simulink model "SimulationDemo_Ship"  (R2025a)
settings: Solver=ode4  StartTime=0.0  StopTime=200  FixedStep=0.02  RelTol=1e-3
InitFcn:
  | Initialization
model workspace (MAT data in the model file):
  actuatorInitial : object (value not decoded)
  contactParams : object (value not decoded)
  flightProtection : object (value not decoded)
  initial : object (value not decoded)
symbols that are objects in the model workspace (value not decoded): actuatorInitial, contactParams, flightProtection, initial
undefined symbols (not defined in the file): aeroData, aileronMax, aileronMin, dirPitch, dirRoll, dirThrottle, dirYaw, elevatorMax, elevatorMin, envCatalog, F, geometry, Light, MIL, pitchCh, pitchDB, propulsionData, rollCh, rollDB, rudderMax, rudderMin, throttleCh, throttleDB, uPitchMax, uPitchMin, uRollMax, uRollMin, uThrottleMax, uThrottleMin, uYawMax, uYawMin, yawCh, yawDB
libraries: simulink_extras x4, aerolibwind2 x3, aerolibasang x2, aerolibsim3d x2, aerolibadyn x1, matrix_library x1, aerolibanimutils x1, aerolibatmos2 x1, uavutilslib x1, sim3dlib x1
(part 2 of 2)

== system SimulationDemo_Ship/Aircraft Dynamics/Forces & Moments/Aerodynamic Forces & Moments/Elevator Contribution ==
  Elevator : Inport
  Alpha : Inport  Port=2
  Bus Creator : BusCreator  Inputs=3
  CD Lookup : Lookup_n-D  LookupTableObject=k  BreakpointsForDimension1=aeroData.elevatorData.ControlDeflections  BreakpointsForDimension2=aeroData.elevatorData.Alpha  Table=aeroData.elevatorData.CD  InternalRulePriority=Speed  RndMeth=Simplest
      settings: InputPortMap=u0,u1
  "CL Lookup " : Lookup_n-D  BreakpointsForDimension1=aeroData.elevatorData.ControlDeflections  BreakpointsForDimension2=aeroData.elevatorData.Alpha  Table=aeroData.elevatorData.CL  InternalRulePriority=Speed  RndMeth=Simplest
      settings: InputPortMap=u0,u1
  Cm Lookup : Lookup_n-D  BreakpointsForDimension1=aeroData.elevatorData.ControlDeflections  BreakpointsForDimension2=aeroData.elevatorData.Alpha  Table=aeroData.elevatorData.Cm  InternalRulePriority=Speed  RndMeth=Simplest
      settings: InputPortMap=u0,u1
  Elevator Contribution : Outport
  wires:
  Bus Creator/1 -> Elevator Contribution/1
  Alpha/1 -> Cm Lookup/2, "CL Lookup "/2, CD Lookup/2
  Elevator/1 -> "CL Lookup "/1, Cm Lookup/1, CD Lookup/1
  Cm Lookup/1 -> Bus Creator/3  "Cm"
  CD Lookup/1 -> Bus Creator/1  "CD"
  "CL Lookup "/1 -> Bus Creator/2  "CL"

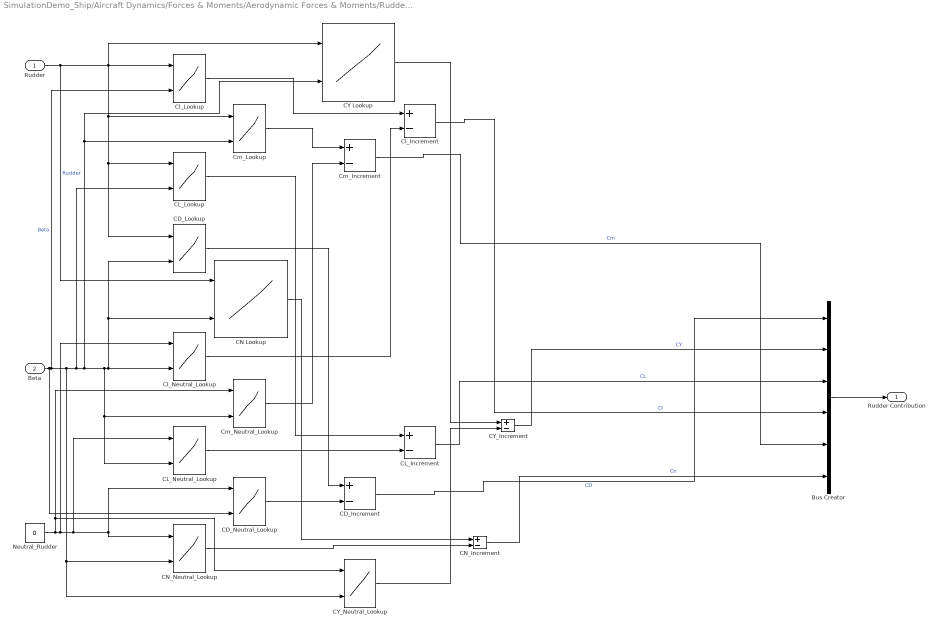
== system SimulationDemo_Ship/Aircraft Dynamics/Forces & Moments/Aerodynamic Forces & Moments/Rudder Contribution ==
  Rudder : Inport
  Beta : Inport  Port=2
  Bus Creator : BusCreator  Inputs=6
  CD_Increment : Sum  Inputs=+-
  CD_Lookup : Lookup_n-D  BreakpointsForDimension1=aeroData.rudderData.ControlDeflections  BreakpointsForDimension2=aeroData.rudderData.Beta  Table=aeroData.rudderData.CD
      settings: InputPortMap=u0,u1
  CD_Neutral_Lookup : Lookup_n-D  BreakpointsForDimension1=aeroData.rudderData.ControlDeflections  BreakpointsForDimension2=aeroData.rudderData.Beta  Table=aeroData.rudderData.CD
      settings: InputPortMap=u0,u1
  CL_Increment : Sum  Inputs=+-
  CL_Lookup : Lookup_n-D  BreakpointsForDimension1=aeroData.rudderData.ControlDeflections  BreakpointsForDimension2=aeroData.rudderData.Beta  Table=aeroData.rudderData.CL
      settings: InputPortMap=u0,u1
  CL_Neutral_Lookup : Lookup_n-D  BreakpointsForDimension1=aeroData.rudderData.ControlDeflections  BreakpointsForDimension2=aeroData.rudderData.Beta  Table=aeroData.rudderData.CL
      settings: InputPortMap=u0,u1
  "CN Lookup " : Lookup_n-D  BreakpointsForDimension1=aeroData.rudderData.ControlDeflections  BreakpointsForDimension2=aeroData.rudderData.Beta  Table=aeroData.rudderData.Cn  InternalRulePriority=Speed  RndMeth=Simplest
      settings: InputPortMap=u0,u1
  CN_Increment : Sum  Inputs=+-
  CN_Neutral_Lookup : Lookup_n-D  BreakpointsForDimension1=aeroData.rudderData.ControlDeflections  BreakpointsForDimension2=aeroData.rudderData.Beta  Table=aeroData.rudderData.Cn
      settings: InputPortMap=u0,u1
  CY Lookup : Lookup_n-D  BreakpointsForDimension1=aeroData.rudderData.ControlDeflections  BreakpointsForDimension2=aeroData.rudderData.Beta  Table=aeroData.rudderData.CY  InternalRulePriority=Speed  RndMeth=Simplest
      settings: InputPortMap=u0,u1
  CY_Increment : Sum  Inputs=+-
  CY_Neutral_Lookup : Lookup_n-D  BreakpointsForDimension1=aeroData.rudderData.ControlDeflections  BreakpointsForDimension2=aeroData.rudderData.Beta  Table=aeroData.rudderData.CY
      settings: InputPortMap=u0,u1
  Cl_Increment : Sum  Inputs=+-
  Cl_Lookup : Lookup_n-D  BreakpointsForDimension1=aeroData.rudderData.ControlDeflections  BreakpointsForDimension2=aeroData.rudderData.Beta  Table=aeroData.rudderData.Cl
      settings: InputPortMap=u0,u1
  Cl_Neutral_Lookup : Lookup_n-D  BreakpointsForDimension1=aeroData.rudderData.ControlDeflections  BreakpointsForDimension2=aeroData.rudderData.Beta  Table=aeroData.rudderData.Cl
      settings: InputPortMap=u0,u1
  Cm_Increment : Sum  Inputs=+-
  Cm_Lookup : Lookup_n-D  BreakpointsForDimension1=aeroData.rudderData.ControlDeflections  BreakpointsForDimension2=aeroData.rudderData.Beta  Table=aeroData.rudderData.Cm
      settings: InputPortMap=u0,u1
  Cm_Neutral_Lookup : Lookup_n-D  BreakpointsForDimension1=aeroData.rudderData.ControlDeflections  BreakpointsForDimension2=aeroData.rudderData.Beta  Table=aeroData.rudderData.Cm
      settings: InputPortMap=u0,u1
  Neutral_Rudder : Constant  Value=0
  "Rudder Contribution " : Outport
  wires:
  Cm_Neutral_Lookup/1 -> Cm_Increment/2
  Cm_Lookup/1 -> Cm_Increment/1
  Cl_Neutral_Lookup/1 -> Cl_Increment/2
  Cl_Lookup/1 -> Cl_Increment/1
  CL_Neutral_Lookup/1 -> CL_Increment/2
  CL_Lookup/1 -> CL_Increment/1
  CD_Neutral_Lookup/1 -> CD_Increment/2
  CD_Lookup/1 -> CD_Increment/1
  Rudder/1 -> CD_Lookup/1, CL_Lookup/1, Cm_Lookup/1, CY Lookup/1, Cl_Lookup/1, "CN Lookup "/1  "Rudder"
  Beta/1 -> CY_Neutral_Lookup/2, CN_Neutral_Lookup/2, CL_Neutral_Lookup/2, Cm_Neutral_Lookup/2, "CN Lookup "/2, CD_Lookup/2, Cl_Neutral_Lookup/2, CY Lookup/2, Cm_Lookup/2, CL_Lookup/2, Cl_Lookup/2, CD_Neutral_Lookup/2  "Beta"
  Neutral_Rudder/1 -> CN_Neutral_Lookup/1, CD_Neutral_Lookup/1, CL_Neutral_Lookup/1, Cl_Neutral_Lookup/1, CY_Neutral_Lookup/1, Cm_Neutral_Lookup/1
  CY Lookup/1 -> CY_Increment/1
  CY_Neutral_Lookup/1 -> CY_Increment/2
  "CN Lookup "/1 -> CN_Increment/1
  CN_Neutral_Lookup/1 -> CN_Increment/2
  Cl_Increment/1 -> Bus Creator/4  "Cl"
  CD_Increment/1 -> Bus Creator/1  "CD"
  Cm_Increment/1 -> Bus Creator/5  "Cm"
  CY_Increment/1 -> Bus Creator/2  "CY"
  CL_Increment/1 -> Bus Creator/3  "CL"
  Bus Creator/1 -> "Rudder Contribution "/1
  CN_Increment/1 -> Bus Creator/6  "Cn"

== system SimulationDemo_Ship/Aircraft Dynamics/Forces & Moments/Aerodynamic Forces & Moments/Subsystem ==
  Elevator contributiotion : Inport
  Aileron contributiotion : Inport  Port=2
  Rudder contributiotion : Inport  Port=3
  Damping rate contributions : Inport  Port=4
  Bus Selector : BusSelector  OutputSignals=CD,CL,Cm
  Bus Selector1 : BusSelector  OutputSignals=CD,CY,CL,Cl,Cm,Cn
  Bus Selector2 : BusSelector  OutputSignals=CD,CY,CL,Cl,Cm,Cn
  Bus Selector3 : BusSelector  OutputSignals=CD_rate,CY_rate,CL_rate,Cl_damp,Cm_damp,Cn_damp
  CD_Total : Sum  Inputs=++++
  CL_Total : Sum  Inputs=++++
  CY_Total : Sum  Inputs=+++
  Cl_Base_Total : Sum  Inputs=+++
  Cm_Base_Total : Sum  Inputs=++++
  Cn_Base_Total : Sum  Inputs=+++
  Moment coefficients : Mux  Inputs=3
  Mux : Mux  Inputs=3
  Forces Coefficients : Outport
  Moment Coefficients : Outport  Port=2
  wires:
  Bus Selector3/2 -> CY_Total/3  "<CY_rate>"
  Bus Selector2/3 -> CL_Total/3  "<CL>"
  Elevator contributiotion/1 -> Bus Selector/1
  CL_Total/1 -> Mux/3  "CL_Total"
  Aileron contributiotion/1 -> Bus Selector1/1
  Cn_Base_Total/1 -> Moment coefficients/3
  Rudder contributiotion/1 -> Bus Selector2/1
  Bus Selector1/1 -> CD_Total/2  "<CD>"
  Damping rate contributions/1 -> Bus Selector3/1
  Bus Selector/1 -> CD_Total/1  "<CD>"
  Bus Selector/2 -> CL_Total/1  "<CL>"
  Bus Selector2/1 -> CD_Total/3  "<CD>"
  Bus Selector/3 -> Cm_Base_Total/1  "<Cm>"
  Bus Selector1/2 -> CY_Total/1  "<CY>"
  CY_Total/1 -> Mux/2  "CY_Total"
  Bus Selector1/3 -> CL_Total/2  "<CL>"
  Bus Selector1/4 -> Cl_Base_Total/1  "<Cl>"
  Bus Selector1/5 -> Cm_Base_Total/2  "<Cm>"
  Mux/1 -> Forces Coefficients/1
  Bus Selector1/6 -> Cn_Base_Total/1  "<Cn>"
  Bus Selector2/2 -> CY_Total/2  "<CY>"
  Bus Selector2/4 -> Cl_Base_Total/2  "<Cl>"
  Bus Selector2/5 -> Cm_Base_Total/3  "<Cm>"
  Bus Selector2/6 -> Cn_Base_Total/2  "<Cn>"
  Bus Selector3/1 -> CD_Total/4  "<CD_rate>"
  Bus Selector3/3 -> CL_Total/4  "<CL_rate>"
  Bus Selector3/4 -> Cl_Base_Total/3  "<Cl_damp>"
  Bus Selector3/5 -> Cm_Base_Total/4  "<Cm_damp>"
  Bus Selector3/6 -> Cn_Base_Total/3  "<Cn_damp>"
  CD_Total/1 -> Mux/1  "CD_Total"
  Cl_Base_Total/1 -> Moment coefficients/1
  Cm_Base_Total/1 -> Moment coefficients/2
  Moment coefficients/1 -> Moment Coefficients/1

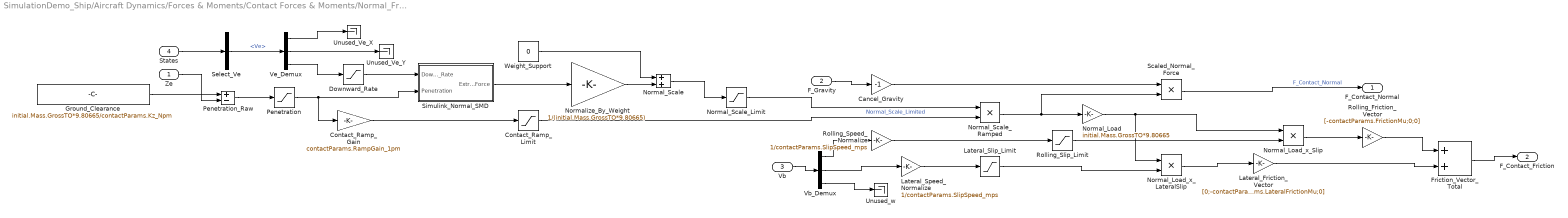
== system SimulationDemo_Ship/Aircraft Dynamics/Forces & Moments/Contact Forces & Moments/Normal_Friction_Forces ==
  Ze : Inport
  F_Gravity : Inport  Port=2
  Vb : Inport  Port=3
  States : Inport  Port=4
  Cancel_Gravity : Gain  Gain=-1
  Contact_Ramp_Gain : Gain  Gain=contactParams.RampGain_1pm
  Contact_Ramp_Limit : Saturate  UpperLimit=1  LowerLimit=0
  Downward_Rate : Saturate  UpperLimit=inf  LowerLimit=-inf
  Friction_Vector_Total : Sum
  Ground_Clearance : Constant  Value=initial.Mass.GrossTO*9.80665/contactParams.Kz_Npm
  Lateral_Friction_Vector : Gain  Gain=[0;-contactParams.LateralFrictionMu;0]
  Lateral_Slip_Limit : Saturate  UpperLimit=1  LowerLimit=-1
  Lateral_Speed_Normalize : Gain  Gain=1/contactParams.SlipSpeed_mps
  Normal_Load : Gain  Gain=initial.Mass.GrossTO*9.80665
  Normal_Load_x_LateralSlip : Product
  Normal_Load_x_Slip : Product
  Normal_Scale : Sum
  Normal_Scale_Limit : Saturate  UpperLimit=contactParams.NormalScaleMax  LowerLimit=0
  Normal_Scale_Ramped : Product
  Normalize_By_Weight : Gain  Gain=1/(initial.Mass.GrossTO*9.80665)
  Penetration : Saturate  UpperLimit=inf  LowerLimit=0
  Penetration_Raw : Sum  Inputs=+-
  Rolling_Friction_Vector : Gain  Gain=[-contactParams.FrictionMu;0;0]
  Rolling_Slip_Limit : Saturate  UpperLimit=1  LowerLimit=-1
  Rolling_Speed_Normalize : Gain  Gain=1/contactParams.SlipSpeed_mps
  Scaled_Normal_Force : Product
  Select_Ve : BusSelector  OutputSignals=Ve
  Simulink_Normal_SMD : Subsystem
  Unused_Ve_X : Terminator
  Unused_Ve_Y : Terminator
  Unused_w : Terminator
  Vb_Demux : Demux  Outputs=3
  Ve_Demux : Demux  Outputs=3
  Weight_Support : Constant  Value=0
  F_Contact_Normal : Outport
  F_Contact_Friction : Outport  Port=2
  wires:
  Friction_Vector_Total/1 -> F_Contact_Friction/1
  Lateral_Friction_Vector/1 -> Friction_Vector_Total/2
  Rolling_Friction_Vector/1 -> Friction_Vector_Total/1
  Normal_Load_x_LateralSlip/1 -> Lateral_Friction_Vector/1
  Lateral_Slip_Limit/1 -> Normal_Load_x_LateralSlip/2
  Lateral_Speed_Normalize/1 -> Lateral_Slip_Limit/1
  Vb_Demux/2 -> Lateral_Speed_Normalize/1
  Normalize_By_Weight/1 -> Normal_Scale/2
  Penetration/1 -> Simulink_Normal_SMD/2(Penetration), Contact_Ramp_Gain/1
  Rolling_Slip_Limit/1 -> Normal_Load_x_Slip/2
  Normal_Scale_Ramped/1 -> Normal_Load/1, Scaled_Normal_Force/2
  Ze/1 -> Penetration_Raw/2
  Contact_Ramp_Limit/1 -> Normal_Scale_Ramped/2
  Ground_Clearance/1 -> Penetration_Raw/1
  Normal_Scale_Limit/1 -> Normal_Scale_Ramped/1  "Normal_Scale_Limited"
  Contact_Ramp_Gain/1 -> Contact_Ramp_Limit/1
  Downward_Rate/1 -> Simulink_Normal_SMD/1(Downward_Rate)
  Penetration_Raw/1 -> Penetration/1
  Scaled_Normal_Force/1 -> F_Contact_Normal/1  "F_Contact_Normal"
  Normal_Load/1 -> Normal_Load_x_Slip/1, Normal_Load_x_LateralSlip/1
  F_Gravity/1 -> Cancel_Gravity/1
  Normal_Scale/1 -> Normal_Scale_Limit/1
  Simulink_Normal_SMD/1(Extra_Normal_Force) -> Normalize_By_Weight/1
  Vb_Demux/1 -> Rolling_Speed_Normalize/1
  Weight_Support/1 -> Normal_Scale/1
  Cancel_Gravity/1 -> Scaled_Normal_Force/1
  Vb/1 -> Vb_Demux/1
  Rolling_Speed_Normalize/1 -> Rolling_Slip_Limit/1
  Normal_Load_x_Slip/1 -> Rolling_Friction_Vector/1
  Vb_Demux/3 -> Unused_w/1
  States/1 -> Select_Ve/1
  Select_Ve/1 -> Ve_Demux/1  "<Ve>"
  Ve_Demux/1 -> Unused_Ve_X/1
  Ve_Demux/2 -> Unused_Ve_Y/1
  Ve_Demux/3 -> Downward_Rate/1

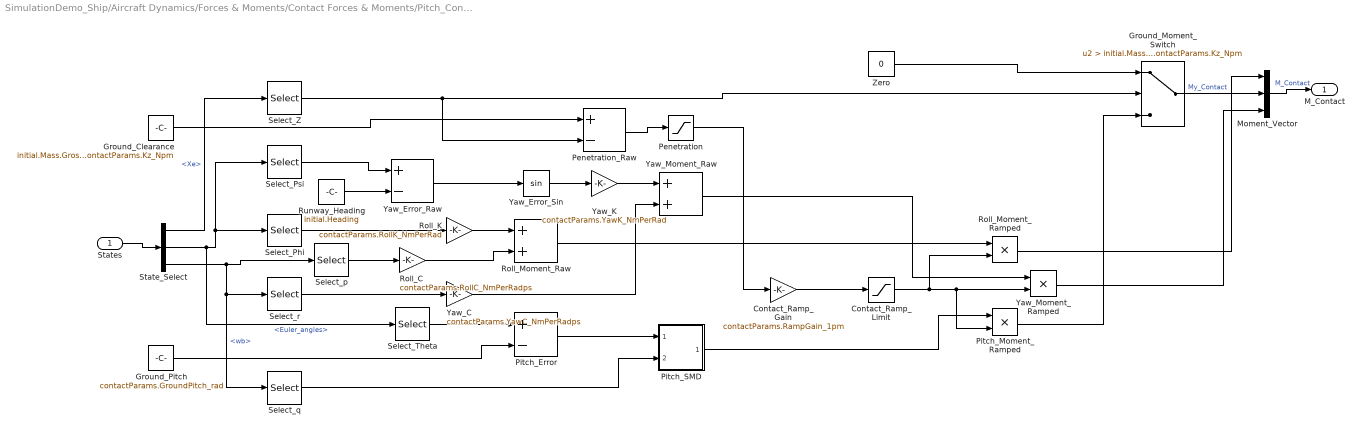
== system SimulationDemo_Ship/Aircraft Dynamics/Forces & Moments/Contact Forces & Moments/Pitch_Contact_Moment ==
  States : Inport
  Contact_Ramp_Gain : Gain  Gain=contactParams.RampGain_1pm
  Contact_Ramp_Limit : Saturate  UpperLimit=1  LowerLimit=0
  Ground_Clearance : Constant  Value=initial.Mass.GrossTO*9.80665/contactParams.Kz_Npm
  Ground_Moment_Switch : Switch  Criteria=u2 > Threshold  Threshold=initial.Mass.GrossTO*9.80665/contactParams.Kz_Npm
  Ground_Pitch : Constant  Value=contactParams.GroundPitch_rad
  Moment_Vector : Mux  Inputs=3
  Penetration : Saturate  UpperLimit=inf  LowerLimit=0
  Penetration_Raw : Sum  Inputs=+-
  Pitch_Error : Sum  Inputs=+-
  Pitch_Moment_Ramped : Product
  Pitch_SMD : Subsystem
  Roll_C : Gain  Gain=contactParams.RollC_NmPerRadps
  Roll_K : Gain  Gain=contactParams.RollK_NmPerRad
  Roll_Moment_Ramped : Product
  Roll_Moment_Raw : Sum
  Runway_Heading : Constant  Value=initial.Heading
  Select_Phi : Selector  InputPortWidth=3  IndexOptions=Index vector (dialog)  Indices=1  OutputSizes=1
  Select_Psi : Selector  InputPortWidth=3  IndexOptions=Index vector (dialog)  Indices=3  OutputSizes=1
  Select_Theta : Selector  InputPortWidth=3  IndexOptions=Index vector (dialog)  Indices=[2]  OutputSizes=1
  Select_Z : Selector  InputPortWidth=3  IndexOptions=Index vector (dialog)  Indices=[3]  OutputSizes=1
  Select_p : Selector  InputPortWidth=3  IndexOptions=Index vector (dialog)  Indices=1  OutputSizes=1
  Select_q : Selector  InputPortWidth=3  IndexOptions=Index vector (dialog)  Indices=[2]  OutputSizes=1
  Select_r : Selector  InputPortWidth=3  IndexOptions=Index vector (dialog)  Indices=3  OutputSizes=1
  State_Select : BusSelector  OutputSignals=Xe,Euler_angles,wb
  Yaw_C : Gain  Gain=contactParams.YawC_NmPerRadps
  Yaw_Error_Raw : Sum  Inputs=+-
  Yaw_Error_Sin : Trigonometry
  Yaw_K : Gain  Gain=contactParams.YawK_NmPerRad
  Yaw_Moment_Ramped : Product
  Yaw_Moment_Raw : Sum
  Zero : Constant  Value=0
  M_Contact : Outport
  wires:
  Yaw_Moment_Ramped/1 -> Moment_Vector/3
  Roll_Moment_Ramped/1 -> Moment_Vector/1
  Yaw_Moment_Raw/1 -> Yaw_Moment_Ramped/1
  Yaw_C/1 -> Yaw_Moment_Raw/2
  Yaw_K/1 -> Yaw_Moment_Raw/1
  Select_r/1 -> Yaw_C/1
  Yaw_Error_Sin/1 -> Yaw_K/1
  Yaw_Error_Raw/1 -> Yaw_Error_Sin/1
  Runway_Heading/1 -> Yaw_Error_Raw/2
  Select_Psi/1 -> Yaw_Error_Raw/1
  Roll_Moment_Raw/1 -> Roll_Moment_Ramped/1
  Roll_C/1 -> Roll_Moment_Raw/2
  Roll_K/1 -> Roll_Moment_Raw/1
  Select_p/1 -> Roll_C/1
  Select_Phi/1 -> Roll_K/1
  States/1 -> State_Select/1
  State_Select/1 -> Select_Z/1  "<Xe>"
  State_Select/2 -> Select_Phi/1, Select_Psi/1, Select_Theta/1  "<Euler_angles>"
  State_Select/3 -> Select_q/1, Select_r/1, Select_p/1  "<wb>"
  Ground_Clearance/1 -> Penetration_Raw/1
  Select_Z/1 -> Ground_Moment_Switch/2, Penetration_Raw/2
  Penetration_Raw/1 -> Penetration/1
  Penetration/1 -> Contact_Ramp_Gain/1
  Contact_Ramp_Gain/1 -> Contact_Ramp_Limit/1
  Select_Theta/1 -> Pitch_Error/1
  Ground_Pitch/1 -> Pitch_Error/2
  Pitch_Error/1 -> Pitch_SMD/1(Pitch_Error)
  Select_q/1 -> Pitch_SMD/2(Pitch_Rate)
  Pitch_SMD/1(Pitch_Moment) -> Pitch_Moment_Ramped/1
  Contact_Ramp_Limit/1 -> Pitch_Moment_Ramped/2, Yaw_Moment_Ramped/2, Roll_Moment_Ramped/2
  Zero/1 -> Ground_Moment_Switch/1
  Pitch_Moment_Ramped/1 -> Ground_Moment_Switch/3
  Ground_Moment_Switch/1 -> Moment_Vector/2  "My_Contact"
  Moment_Vector/1 -> M_Contact/1  "M_Contact"

== system SimulationDemo_Ship/Aircraft Dynamics/Forces & Moments/Propulsion Forces & Moments/Density Correction ==
  In1 : Inport
  Bus Selector1 : BusSelector  OutputSignals=rho
  Constant : Constant  Value=1.225
  Divide : Product  Inputs=*/
  Out1 : Outport
  wires:
  Bus Selector1/1 -> Divide/1  "<rho>"
  Divide/1 -> Out1/1
  Constant/1 -> Divide/2
  In1/1 -> Bus Selector1/1

== system SimulationDemo_Ship/Aircraft Dynamics/Forces & Moments/Propulsion Forces & Moments/Subsystem ==
  Forces : Inport
  Cross Product : matrix_library/Cross Product
  Position Vector : Concatenate  NumInputs=3  ConcatenateDimension=2
  Thrust Vector : Concatenate  NumInputs=1  Mode=Multidimensional array  ConcatenateDimension=3
  rX : Constant  Value=geometry.PropArmX
  rY : Constant  Value=geometry.PropArmY
  rZ : Constant  Value=geometry.PropArmZ
  Moments : Outport
  wires:
  rZ/1 -> Position Vector/3
  rY/1 -> Position Vector/2
  rX/1 -> Position Vector/1
  Forces/1 -> Thrust Vector/1
  Cross Product/1 -> Moments/1
  Position Vector/1 -> Cross Product/1
  Thrust Vector/1 -> Cross Product/2

== system SimulationDemo_Ship/Aircraft Dynamics/Forces & Moments/Propulsion Forces & Moments/Subsystem1 ==
  Density corrected Thrust : Inport
  Constant : Constant  Value=0
  Cos : Trigonometry  Operator=cos
  Gain : Gain  Gain=-1
  Mux : Mux  Inputs=3
  Product : Product
  Product1 : Product
  Sin : Trigonometry
  Thrust Incidence : Constant  Value=geometry.ThrustIncidence_deg*pi/180
  Forces_Propulsion : Outport
  wires:
  Gain/1 -> Mux/3  "Thrust Z"
  Cos/1 -> Product/2
  Product/1 -> Mux/1  "Thrust X"
  Density corrected Thrust/1 -> Product1/1, Product/1
  Thrust Incidence/1 -> Sin/1, Cos/1
  Sin/1 -> Product1/2
  Product1/1 -> Gain/1
  Constant/1 -> Mux/2  "Thrust Y"
  Mux/1 -> Forces_Propulsion/1  "Forces_Propulsion"

== system SimulationDemo_Ship/Aircraft Dynamics/Forces & Moments/Propulsion Forces & Moments/Subsystem2 ==
  Pilot_Inputs : Inport
  Bus Selector : BusSelector  OutputSignals=Throttle
  Inv_Thrust_Tau : Gain  Gain=5
  Thrust : Lookup_n-D  NumberOfTableDimensions=1  BreakpointsForDimension1=propulsionData.Throttle  IndexSearchMethod=Evenly spaced points  Table=propulsionData.Thrust_Newtons  InternalRulePriority=Speed  RndMeth=Simplest
  Thrust_Lag : Integrator
  Thrust_Lag_Error : Sum  Inputs=+-
  Thrust_Rate_Limiter : RateLimiter  RisingSlewLimit=max(propulsionData.Thrust_Newtons(:))/0.2  FallingSlewLimit=-max(propulsionData.Thrust_Newtons(:))/0.2
  Motor_Prop_Thrust : Outport
  wires:
  Bus Selector/1 -> Thrust/1  "<Throttle>"
  Inv_Thrust_Tau/1 -> Thrust_Lag/1
  Thrust_Lag_Error/1 -> Inv_Thrust_Tau/1
  Thrust_Lag/1 -> Thrust_Lag_Error/2, Motor_Prop_Thrust/1  "Motor_Prop_Thrust"
  Pilot_Inputs/1 -> Bus Selector/1
  Thrust/1 -> Thrust_Rate_Limiter/1  "Static_Thrust"
  Thrust_Rate_Limiter/1 -> Thrust_Lag_Error/1  "Rate_Limited_Thrust"

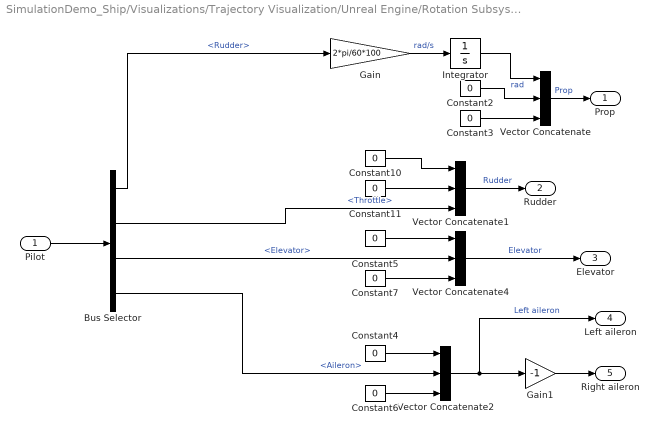
== system SimulationDemo_Ship/Visualizations/Trajectory Visualization/Unreal Engine/Rotation Subsystem ==
  Pilot : Inport
  Bus Selector : BusSelector  OutputSignals=Rudder,Throttle,Elevator,Aileron
  Constant{2..7,10..11} (8 alike) : Constant  Value=0
  Gain : Gain  Gain=2*pi/60*100
  Gain1 : Gain  Gain=-1
  Integrator : Integrator
  Vector Concatenate{,1..2,4} (4 alike) : Concatenate  NumInputs=3  Mode=Multidimensional array  ConcatenateDimension=2
  Prop : Outport  Unit=rad  PortDimensions=[1,3]
  Rudder : Outport  Port=2  Unit=rad  PortDimensions=[1,3]
  Elevator : Outport  Port=3  Unit=rad  PortDimensions=[1,3]
  Left aileron : Outport  Port=4  Unit=rad  PortDimensions=[1,3]
  Right aileron : Outport  Port=5  Unit=rad  PortDimensions=[1,3]
  wires:
  Constant6/1 -> Vector Concatenate2/3
  Constant4/1 -> Vector Concatenate2/1
  Gain1/1 -> Right aileron/1
  Constant11/1 -> Vector Concatenate1/2
  Constant10/1 -> Vector Concatenate1/1
  Constant5/1 -> Vector Concatenate4/1
  Pilot/1 -> Bus Selector/1
  Bus Selector/2 -> Vector Concatenate1/3  "<Throttle>"
  Constant3/1 -> Vector Concatenate/3
  Bus Selector/4 -> Vector Concatenate2/2  "<Aileron>"
  Bus Selector/3 -> Vector Concatenate4/2  "<Elevator>"
  Bus Selector/1 -> Gain/1  "<Rudder>"
  Constant7/1 -> Vector Concatenate4/3
  Vector Concatenate1/1 -> Rudder/1  "Rudder"
  Integrator/1 -> Vector Concatenate/1  "rad"
  Vector Concatenate2/1 -> Gain1/1, Left aileron/1  "Left aileron"
  Vector Concatenate4/1 -> Elevator/1  "Elevator"
  Gain/1 -> Integrator/1  "rad/s"
  Constant2/1 -> Vector Concatenate/2
  Vector Concatenate/1 -> Prop/1  "Prop"

== system SimulationDemo_Ship/Aircraft Dynamics/Forces & Moments/Aerodynamic Forces & Moments/Damping rate coefficients/Cl ==
  p_nd : Inport
  beta : Inport  Port=2
  r_nd : Inport  Port=3
  Constant : Constant  Value=aeroData.stabilityDerivatives.Clp
  Constant1 : Constant  Value=aeroData.stabilityDerivatives.Clr
  Constant2 : Constant  Value=aeroData.stabilityDerivatives.Clb
  Product : Product
  Product1 : Product
  Product2 : Product
  Sum : Sum  Inputs=|+++
  Cl_damp : Outport  VectorParamsAs1DForOutWhenUnconnected=off
  wires:
  Product2/1 -> Sum/3
  Product/1 -> Sum/1
  Constant/1 -> Product/1
  Constant2/1 -> Product1/1
  p_nd/1 -> Product/2
  beta/1 -> Product1/2
  Product1/1 -> Sum/2
  Constant1/1 -> Product2/1
  Sum/1 -> Cl_damp/1
  r_nd/1 -> Product2/2

== system SimulationDemo_Ship/Aircraft Dynamics/Forces & Moments/Aerodynamic Forces & Moments/Damping rate coefficients/Cm ==
  q_nd : Inport
  Constant : Constant  Value=aeroData.stabilityDerivatives.Cmq
  Product : Product
  Cm_damp : Outport
  wires:
  Constant/1 -> Product/1
  q_nd/1 -> Product/2
  Product/1 -> Cm_damp/1  "Cm_damp"

== system SimulationDemo_Ship/Aircraft Dynamics/Forces & Moments/Aerodynamic Forces & Moments/Damping rate coefficients/Cn ==
  p_nd : Inport
  beta : Inport  Port=2
  r_nd : Inport  Port=3
  Constant : Constant  Value=aeroData.stabilityDerivatives.Cnp
  Constant1 : Constant  Value=aeroData.stabilityDerivatives.Cnr
  Constant2 : Constant  Value=aeroData.stabilityDerivatives.Cnb
  Product : Product
  Product1 : Product
  Product2 : Product
  Sum : Sum  Inputs=|+++
  Cn_damp : Outport  VectorParamsAs1DForOutWhenUnconnected=off
  wires:
  r_nd/1 -> Product2/2
  Constant1/1 -> Product2/1
  Constant2/1 -> Product1/1
  Constant/1 -> Product/1
  p_nd/1 -> Product/2
  beta/1 -> Product1/2
  Product1/1 -> Sum/2
  Product/1 -> Sum/1
  Product2/1 -> Sum/3
  Sum/1 -> Cn_damp/1

== system SimulationDemo_Ship/Aircraft Dynamics/Forces & Moments/Aerodynamic Forces & Moments/Damping rate coefficients/Non Dimensionalize p,q,r ==
  note: Note: VMin is used to avoid singluraties that may arise due to 1/V_TAS
  p,q,r : Inport  Unit=rad/second
  V_TAS : Inport  Port=2  Unit=m/second
  Demux : Demux  Outputs=3
      settings: DisplayOption=none
  Divide : Product  Inputs=*/
  Divide1 : Product  Inputs=*/
  Divide2 : Product  Inputs=*/
  Gain : Gain  Gain=geometry.Span
  Gain1 : Gain  Gain=geometry.Span
  Gain2 : Gain  Gain=geometry.MAC
  Gain3 : Gain  Gain=2
  Max : MinMax  Function=max  Inputs=2
  VMin : Constant  Value=flightProtection.VMin_mps
  p_nd : Outport
  q_nd : Outport  Port=2
  r_nd : Outport  Port=3
  wires:
  Demux/3 -> Divide2/1  "r"
  V_TAS/1 -> Gain3/1
  Gain3/1 -> Max/1
  Demux/1 -> Divide/1  "p"
  Gain2/1 -> q_nd/1
  Divide2/1 -> Gain1/1
  Divide/1 -> Gain/1
  Demux/2 -> Divide1/1  "q"
  p,q,r/1 -> Demux/1
  Divide1/1 -> Gain2/1
  Gain1/1 -> r_nd/1
  Gain/1 -> p_nd/1
  VMin/1 -> Max/2
  Max/1 -> Divide2/2, Divide/2, Divide1/2  "V_TAS_Safe"

== system SimulationDemo_Ship/Aircraft Dynamics/Forces & Moments/Contact Forces & Moments/Normal_Friction_Forces/Simulink_Normal_SMD ==
  Downward_Rate : Inport
  Penetration : Inport  Port=2
  Add_Force : Sum  Inputs=|++
  Damper_C : Gain  Gain=contactParams.Cz_Nspm
  Spring_K : Gain  Gain=contactParams.Kz_Npm
  Extra_Normal_Force : Outport
  wires:
  Add_Force/1 -> Extra_Normal_Force/1
  Damper_C/1 -> Add_Force/2
  Spring_K/1 -> Add_Force/1
  Downward_Rate/1 -> Damper_C/1
  Penetration/1 -> Spring_K/1

== system SimulationDemo_Ship/Aircraft Dynamics/Forces & Moments/Contact Forces & Moments/Pitch_Contact_Moment/Pitch_SMD ==
  Pitch_Error : Inport
  Pitch_Rate : Inport  Port=2
  Add_Moment : Sum  Inputs=|++
  Pitch_C : Gain  Gain=contactParams.PitchC_NmPerRadps
  Pitch_K : Gain  Gain=contactParams.PitchK_NmPerRad
  Pitch_Moment : Outport
  wires:
  Add_Moment/1 -> Pitch_Moment/1
  Pitch_C/1 -> Add_Moment/2
  Pitch_K/1 -> Add_Moment/1
  Pitch_Rate/1 -> Pitch_C/1
  Pitch_Error/1 -> Pitch_K/1
